simulink model "Simple_3_Model"  (R2022a)
settings: Solver=FixedStepAuto  StartTime=0.0  StopTime=10  FixedStep=.01  RelTol=1e-3
undefined symbols (not defined in the file or in its folder): importedData, robot_Volume, robotCoB, robotCoM, robotMoI, robotPitchDragCoefficients, robotRollDragCoefficients, robotXDragCoefficients, robotYawDragCoefficients, robotYDragCoefficients, robotZDragCoefficients
libraries: matrix_library x9, realtime_pacer_lib x1, ros2lib x1
settings Model: Creator=hollis  LastModifiedBy=hollis

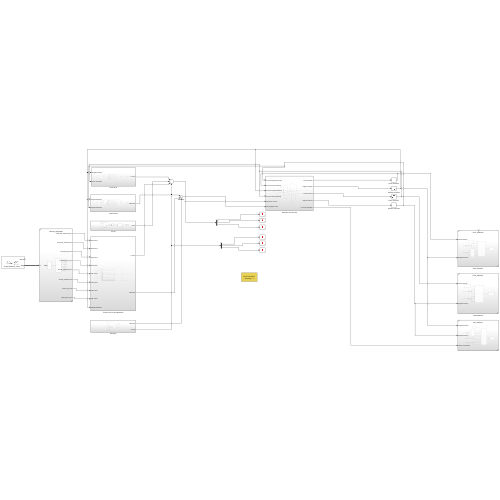
[thumbnail: Simulink's stored preview of the top-level diagram]
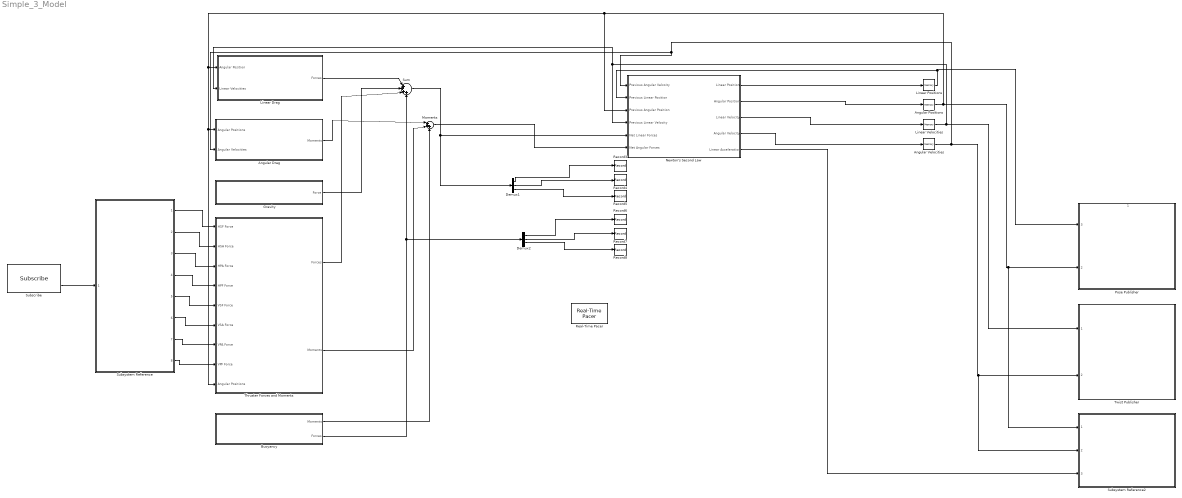
== system Simple_3_Model ==
  Angular Drag : Subsystem
  Angular Positions : Memory
  Angular Velocities : Memory
  Buoyancy : Subsystem
  Demux1 : Demux  Outputs=3
  Demux2 : Demux  Outputs=3
  Gravity : Subsystem
  Linear Drag : Subsystem
  Linear Positions : Memory
  Linear Velocities : Memory
  Moments : Sum  Inputs=|+++
  Newton's Second Law : Subsystem
  Pose Publisher : Subsystem  ReferencedSubsystem=Pose_Publisher
      settings: PortSchema="{\"entries\":[{\"content\":{\"sides\":[{\"content\":{\"connectorIds\":[\"In3\",\"In2\"]},\"type\":\"ConnectorPlacement.EquallySpacedRectSide\",\"uuid\":\"18965d15-4955-4736-88eb-98a03933ea40\"},{\"content\":{\"connectorIds\":[],\"side\":\"RIGHT\"},\"type\":\"ConnectorPlacement.EquallySpacedRectSide\",\"uuid\":\"0239975c-7916-4f79-8798-13edb7247875\"},{\"content\":{\"connectorIds\":[\"In1\"],\"side\":\"TOP\"},\"type\":\"ConnectorPlacement.EquallySpacedRectSide\",\"uuid\":\"c7399201-5872-4101-b484-2a6e35d6576e\"}]},\"type\":\"ConnectorPlacement.EquallySpacedConnector\",\"uuid\":\"5ae7f81e-60af-4dbc-8d3d-d59049f94250\"}],\"packageUris\":[\"http://schema.mathworks.com/mf0/Connector/R2020b\"],\"version\":\"1.0\"}"
  Real-Time Pacer : realtime_pacer_lib/Real-Time Pacer  simTimePerRealTime=1
      settings: SourceProductName=Real-Time Pacer
  Record3 : Record  FileSettingsInternal="{\"entries\":[{\"content\":{\"excelSettings\":{\"content\":{},\"type\":\"Streamout.ExcelSettings\"}},\"type\":\"Streamout.FileSettingStorage\",\"uuid\":\"7fd3eebb-0f88-428b-bc5a-be43bf9f2e21\"}],\"packageUris\":[\"http://schema.mathworks.com/mf0/streamout_blocks/R2020a\"],\"version\":\"1.0\"}"  SignalsInternal="{\"entries\":[{\"content\":{\"signals\":[{\"content\":{\"blockPath\":[\"Simple_3_Model/Record3\"],\"channel\":[],\"dimensions\":[1,1],\"domain\":\"Simple_3_Model/Record3\",\"lineColor\":\"#4dbeee\",\"plots\":[1],\"port\":1,\"sid\":[\"\"],\"signalID\":351,\"signalName\":\"Demux1:1\"},\"type\":\"RecordBlkView.Signal\",\"uuid\":\"b88f4a68-92d4-4a9b-a347-9b0300d270aa\"}]},\"type\":\"RecordBlkView.InputSignals\",\"uuid\":\"525ea289-2c7b-4200-a763-2aaae37b50f9\"}],\"packageUris\":[\"http://schema.mathworks.com/mf0/streamout_blocks/R2020a\"],\"version\":\"1.0\"}"  VisualizationBindings="{\"sparklinesplugin\":{\"info\":[{\"bindingParametersList\":[],\"subplotID\":1}]}}"
  Record4 : Record  FileSettingsInternal="{\"entries\":[{\"content\":{\"excelSettings\":{\"content\":{},\"type\":\"Streamout.ExcelSettings\"}},\"type\":\"Streamout.FileSettingStorage\",\"uuid\":\"25a64ef7-4cd6-46f5-99bd-b94f42d1ee70\"}],\"packageUris\":[\"http://schema.mathworks.com/mf0/streamout_blocks/R2020a\"],\"version\":\"1.0\"}"  SignalsInternal="{\"entries\":[{\"content\":{\"signals\":[{\"content\":{\"blockPath\":[\"Simple_3_Model/Record4\"],\"channel\":[],\"dimensions\":[1,1],\"domain\":\"Simple_3_Model/Record4\",\"lineColor\":\"#a2142f\",\"plots\":[1],\"port\":1,\"sid\":[\"\"],\"signalID\":355,\"signalName\":\"Demux1:2\"},\"type\":\"RecordBlkView.Signal\",\"uuid\":\"ab564040-d490-4015-8163-6bd6843044f3\"}]},\"type\":\"RecordBlkView.InputSignals\",\"uuid\":\"276f9bd8-9c59-4519-84f4-c5845e1178bb\"}],\"packageUris\":[\"http://schema.mathworks.com/mf0/streamout_blocks/R2020a\"],\"version\":\"1.0\"}"  VisualizationBindings="{\"sparklinesplugin\":{\"info\":[{\"bindingParametersList\":[],\"subplotID\":1}]}}"
  Record5 : Record  FileSettingsInternal="{\"entries\":[{\"content\":{\"excelSettings\":{\"content\":{},\"type\":\"Streamout.ExcelSettings\"}},\"type\":\"Streamout.FileSettingStorage\",\"uuid\":\"6c523934-be1b-4723-a5da-1a53bd07d317\"}],\"packageUris\":[\"http://schema.mathworks.com/mf0/streamout_blocks/R2020a\"],\"version\":\"1.0\"}"  SignalsInternal="{\"entries\":[{\"content\":{\"signals\":[{\"content\":{\"blockPath\":[\"Simple_3_Model/Record5\"],\"channel\":[],\"dimensions\":[1,1],\"domain\":\"Simple_3_Model/Record5\",\"lineColor\":\"#139fff\",\"plots\":[1],\"port\":1,\"sid\":[\"\"],\"signalID\":359,\"signalName\":\"Demux1:3\"},\"type\":\"RecordBlkView.Signal\",\"uuid\":\"c0e7c173-a5c9-49b7-9f71-2d8dfa5ec17e\"}]},\"type\":\"RecordBlkView.InputSignals\",\"uuid\":\"c924540a-dae3-4e11-a7aa-2d2acfbdbe16\"}],\"packageUris\":[\"http://schema.mathworks.com/mf0/streamout_blocks/R2020a\"],\"version\":\"1.0\"}"  VisualizationBindings="{\"sparklinesplugin\":{\"info\":[{\"bindingParametersList\":[],\"subplotID\":1}]}}"
  Record6 : Record  FileSettingsInternal="{\"entries\":[{\"content\":{\"excelSettings\":{\"content\":{},\"type\":\"Streamout.ExcelSettings\"}},\"type\":\"Streamout.FileSettingStorage\",\"uuid\":\"7e9df886-1170-419d-9cbc-cbe48d003bf2\"}],\"packageUris\":[\"http://schema.mathworks.com/mf0/streamout_blocks/R2020a\"],\"version\":\"1.0\"}"  SignalsInternal="{\"entries\":[{\"content\":{\"signals\":[{\"content\":{\"blockPath\":[\"Simple_3_Model/Record6\"],\"channel\":[],\"dimensions\":[1,1],\"domain\":\"Simple_3_Model/Record6\",\"lineColor\":\"#edb120\",\"plots\":[1],\"port\":1,\"sid\":[\"\"],\"signalID\":363,\"signalName\":\"Demux2:1\"},\"type\":\"RecordBlkView.Signal\",\"uuid\":\"9d71cc72-7893-4320-bde5-368aaa6a6399\"}]},\"type\":\"RecordBlkView.InputSignals\",\"uuid\":\"6ba886b7-fc5d-4a52-a6dc-8621a5dc22ea\"}],\"packageUris\":[\"http://schema.mathworks.com/mf0/streamout_blocks/R2020a\"],\"version\":\"1.0\"}"  VisualizationBindings="{\"sparklinesplugin\":{\"info\":[{\"bindingParametersList\":[],\"subplotID\":1}]}}"
  Record7 : Record  FileSettingsInternal="{\"entries\":[{\"content\":{\"excelSettings\":{\"content\":{},\"type\":\"Streamout.ExcelSettings\"}},\"type\":\"Streamout.FileSettingStorage\",\"uuid\":\"db813548-beb3-4592-95ed-07357187fff0\"}],\"packageUris\":[\"http://schema.mathworks.com/mf0/streamout_blocks/R2020a\"],\"version\":\"1.0\"}"  SignalsInternal="{\"entries\":[{\"content\":{\"signals\":[{\"content\":{\"blockPath\":[\"Simple_3_Model/Record7\"],\"channel\":[],\"dimensions\":[1,1],\"domain\":\"Simple_3_Model/Record7\",\"lineColor\":\"#7e2f8e\",\"plots\":[1],\"port\":1,\"sid\":[\"\"],\"signalID\":367,\"signalName\":\"Demux2:2\"},\"type\":\"RecordBlkView.Signal\",\"uuid\":\"a9a06697-73f9-436b-bc11-ccf928b186fe\"}]},\"type\":\"RecordBlkView.InputSignals\",\"uuid\":\"18b6c55c-c8ab-460b-beea-45484844a1c5\"}],\"packageUris\":[\"http://schema.mathworks.com/mf0/streamout_blocks/R2020a\"],\"version\":\"1.0\"}"  VisualizationBindings="{\"sparklinesplugin\":{\"info\":[{\"bindingParametersList\":[],\"subplotID\":1}]}}"
  Record8 : Record  FileSettingsInternal="{\"entries\":[{\"content\":{\"excelSettings\":{\"content\":{},\"type\":\"Streamout.ExcelSettings\"}},\"type\":\"Streamout.FileSettingStorage\",\"uuid\":\"193b8698-55d3-4337-bca1-470059843305\"}],\"packageUris\":[\"http://schema.mathworks.com/mf0/streamout_blocks/R2020a\"],\"version\":\"1.0\"}"  SignalsInternal="{\"entries\":[{\"content\":{\"signals\":[{\"content\":{\"blockPath\":[\"Simple_3_Model/Record8\"],\"channel\":[],\"dimensions\":[1,1],\"domain\":\"Simple_3_Model/Record8\",\"lineColor\":\"#77ac30\",\"plots\":[1],\"port\":1,\"sid\":[\"\"],\"signalID\":371,\"signalName\":\"Demux2:3\"},\"type\":\"RecordBlkView.Signal\",\"uuid\":\"1c0420e5-8b4b-4d3a-992d-29d5925925d9\"}]},\"type\":\"RecordBlkView.InputSignals\",\"uuid\":\"2ac1f8f1-2e48-4e86-bbdb-ec48a12e78c2\"}],\"packageUris\":[\"http://schema.mathworks.com/mf0/streamout_blocks/R2020a\"],\"version\":\"1.0\"}"  VisualizationBindings="{\"sparklinesplugin\":{\"info\":[{\"bindingParametersList\":[],\"subplotID\":1}]}}"
  Subscribe : ros2lib/Subscribe  topicSource=Select from ROS network  topic=/tempest/thruster_forces  messageType=std_msgs/Float32MultiArray  sampleTime=-1  QOSHistory=Keep last  QOSDepth=1  QOSReliability=Reliable  QOSDurability=Volatile
      settings: SourceProductBaseCode=RR
  Subsystem Reference : Subsystem  ReferencedSubsystem=Thruster_Magnitude
  Subsystem Reference2 : Subsystem  ReferencedSubsystem=Imu_Publisher
  Sum : Sum  Inputs=|++++
  Thruster Forces and Moments : Subsystem
  Twist Publisher : Subsystem  ReferencedSubsystem=Twist_Publisher
  wires:
  Linear Drag/1(Forces) -> Sum/1
  Gravity/1(Force) -> Sum/2
  Angular Drag/1(Moments) -> Moments/1
  Thruster Forces and Moments/2(Moments) -> Moments/2
  Buoyancy/1(Moments) -> Moments/3
  Angular Velocities/1 -> Subsystem Reference2/2, Twist Publisher/2, Angular Drag/2(Angular Velocities), Newton's Second Law/1(Previous Angular Velcoity)
  Linear Positions/1 -> Pose Publisher/3, Newton's Second Law/2(Previous Linear Position)
  Linear Velocities/1 -> Linear Drag/2(Linear Velocities), Newton's Second Law/4(Previous Linear Velocity), Twist Publisher/1
  Sum/1 -> Demux1/1, Newton's Second Law/5(Net Linear Forces)
  Moments/1 -> Newton's Second Law/6(Net Angular Forces)
  Newton's Second Law/1(Linear Position) -> Linear Positions/1
  Newton's Second Law/2(Angular Position) -> Angular Positions/1
  Newton's Second Law/4(Angular Velocity) -> Angular Velocities/1
  Newton's Second Law/3(Linear Velocity) -> Linear Velocities/1
  Angular Positions/1 -> Linear Drag/1(Angular Position), Thruster Forces and Moments/9(Angular Positions), Angular Drag/1(Angular Positions), Newton's Second Law/3(Previous Angular Position), Subsystem Reference2/1, Pose Publisher/2
  Demux1/2 -> Record4/1
  Demux1/1 -> Record3/1
  Demux1/3 -> Record5/1
  Thruster Forces and Moments/1(Forces) -> Sum/3
  Demux2/2 -> Record7/1
  Demux2/1 -> Record6/1
  Demux2/3 -> Record8/1
  Buoyancy/2(Forces) -> Sum/4, Demux2/1
  Subsystem Reference/1 -> Thruster Forces and Moments/1(HSF Force)
  Subsystem Reference/2 -> Thruster Forces and Moments/2(HSA Force)
  Subsystem Reference/3 -> Thruster Forces and Moments/3(HPA Force)
  Subsystem Reference/4 -> Thruster Forces and Moments/4(HPF Force)
  Subsystem Reference/5 -> Thruster Forces and Moments/5(VSF Force)
  Subsystem Reference/6 -> Thruster Forces and Moments/6(VSA Force)
  Subsystem Reference/7 -> Thruster Forces and Moments/7(VPA Force)
  Subsystem Reference/8 -> Thruster Forces and Moments/8(VPF Force)
  Subscribe/2 -> Subsystem Reference/1
  Newton's Second Law/5(Linear Acceleration) -> Subsystem Reference2/3

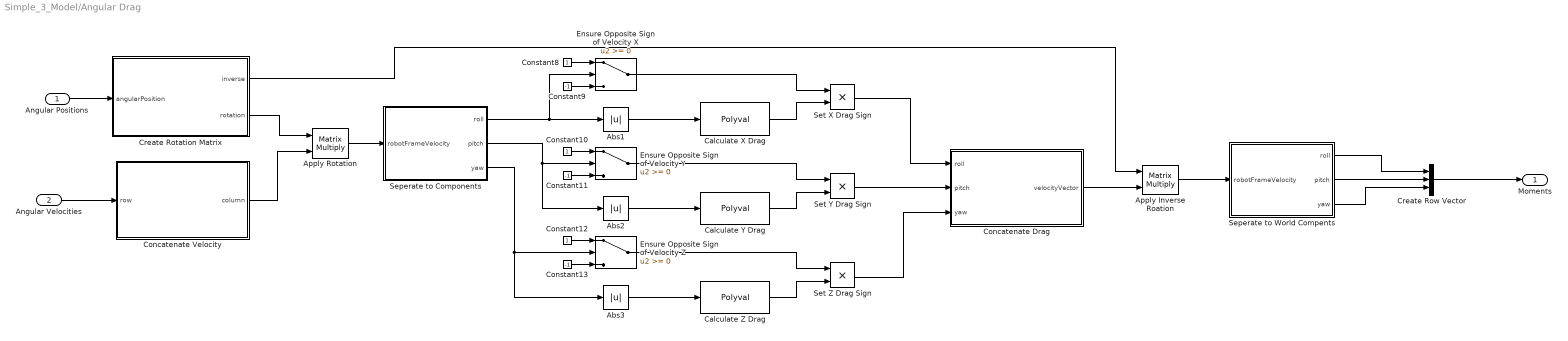
== system Simple_3_Model/Angular Drag ==
  Angular Positions : Inport
  Angular Velocities : Inport  Port=2
  Abs1 : Abs  SaturateOnIntegerOverflow=off
  Abs2 : Abs  SaturateOnIntegerOverflow=off
  Abs3 : Abs  SaturateOnIntegerOverflow=off
  Apply Inverse Roation : Product  Multiplication=Matrix(*)
  Apply Rotation : Product  Multiplication=Matrix(*)
  Calculate X Drag : Polyval  Coefs=robotRollDragCoefficients
  Calculate Y Drag : Polyval  Coefs=robotPitchDragCoefficients
  Calculate Z Drag : Polyval  Coefs=robotYawDragCoefficients
  Concatenate Drag : MATLAB Function  TreatAsAtomicUnit=on
  Concatenate Velocity : MATLAB Function  TreatAsAtomicUnit=on
  Constant10 : Constant
  Constant11 : Constant  Value=-1
  Constant12 : Constant
  Constant13 : Constant  Value=-1
  Constant8 : Constant
  Constant9 : Constant  Value=-1
  Create Rotation Matrix : MATLAB Function  TreatAsAtomicUnit=on
  Create Row Vector : Mux  Inputs=3
  Ensure Opposite Sign of Velocity X : Switch  SaturateOnIntegerOverflow=off  InputSameDT=off
  Ensure Opposite Sign of Velocity Y : Switch  SaturateOnIntegerOverflow=off  InputSameDT=off
  Ensure Opposite Sign of Velocity Z : Switch  SaturateOnIntegerOverflow=off  InputSameDT=off
  Seperate to Components : MATLAB Function  TreatAsAtomicUnit=on
  Seperate to World Compents : MATLAB Function  TreatAsAtomicUnit=on
  Set X Drag Sign : Product
  Set Y Drag Sign : Product
  Set Z Drag Sign : Product
  Moments : Outport
  wires:
  Concatenate Drag/1(velocityVector) -> Apply Inverse Roation/2
  Calculate Y Drag/1 -> Set Y Drag Sign/2
  Constant11/1 -> Ensure Opposite Sign of Velocity Y/3
  Calculate Z Drag/1 -> Set Z Drag Sign/2
  Abs1/1 -> Calculate X Drag/1
  Apply Rotation/1 -> Seperate to Components/1(robotFrameVelocity)
  Apply Inverse Roation/1 -> Seperate to World Compents/1(robotFrameVelocity)
  Angular Velocities/1 -> Concatenate Velocity/1(row)
  Constant8/1 -> Ensure Opposite Sign of Velocity X/1
  Set Z Drag Sign/1 -> Concatenate Drag/3(yaw)
  Constant13/1 -> Ensure Opposite Sign of Velocity Z/3
  Constant9/1 -> Ensure Opposite Sign of Velocity X/3
  Set Y Drag Sign/1 -> Concatenate Drag/2(pitch)
  Ensure Opposite Sign of Velocity Y/1 -> Set Y Drag Sign/1
  Seperate to Components/2(pitch) -> Abs2/1, Ensure Opposite Sign of Velocity Y/2
  Set X Drag Sign/1 -> Concatenate Drag/1(roll)
  Seperate to World Compents/3(yaw) -> Create Row Vector/3
  Constant12/1 -> Ensure Opposite Sign of Velocity Z/1
  Create Rotation Matrix/2(rotation) -> Apply Rotation/1
  Concatenate Velocity/1(column) -> Apply Rotation/2
  Seperate to World Compents/1(roll) -> Create Row Vector/1
  Ensure Opposite Sign of Velocity X/1 -> Set X Drag Sign/1
  Seperate to Components/1(roll) -> Ensure Opposite Sign of Velocity X/2, Abs1/1
  Seperate to World Compents/2(pitch) -> Create Row Vector/2
  Create Rotation Matrix/1(inverse) -> Apply Inverse Roation/1
  Constant10/1 -> Ensure Opposite Sign of Velocity Y/1
  Calculate X Drag/1 -> Set X Drag Sign/2
  Abs2/1 -> Calculate Y Drag/1
  Abs3/1 -> Calculate Z Drag/1
  Seperate to Components/3(yaw) -> Ensure Opposite Sign of Velocity Z/2, Abs3/1
  Ensure Opposite Sign of Velocity Z/1 -> Set Z Drag Sign/1
  Create Row Vector/1 -> Moments/1
  Angular Positions/1 -> Create Rotation Matrix/1(angularPosition)

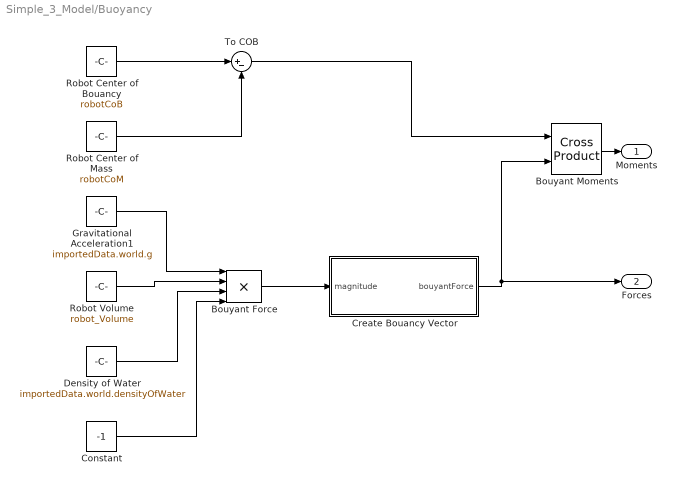
== system Simple_3_Model/Buoyancy ==
  Bouyant Force : Product  Inputs=4
  Bouyant Moments : matrix_library/Cross Product
      settings: SourceProductBaseCode=SL
  Constant : Constant  Value=-1
  Create Bouancy Vector : MATLAB Function  TreatAsAtomicUnit=on
  Density of Water : Constant  Value=importedData.world.densityOfWater
  Gravitational Acceleration1 : Constant  Value=importedData.world.g
  Robot Center of Bouancy : Constant  Value=robotCoB
  Robot Center of Mass : Constant  Value=robotCoM
  Robot Volume : Constant  Value=robot_Volume
  To COB : Sum  Inputs=|+-
  Moments : Outport
  Forces : Outport  Port=2
  wires:
  Density of Water/1 -> Bouyant Force/3
  Gravitational Acceleration1/1 -> Bouyant Force/1
  Robot Center of Bouancy/1 -> To COB/1
  To COB/1 -> Bouyant Moments/1
  Bouyant Force/1 -> Create Bouancy Vector/1(magnitude)
  Create Bouancy Vector/1(bouyantForce) -> Bouyant Moments/2, Forces/1
  Robot Volume/1 -> Bouyant Force/2
  Robot Center of Mass/1 -> To COB/2
  Bouyant Moments/1 -> Moments/1
  Constant/1 -> Bouyant Force/4

== system Simple_3_Model/Gravity ==
  Create Vector : MATLAB Function  TreatAsAtomicUnit=on
  Gravitational Acceleration1 : Constant  Value=importedData.world.g
  Gravitational Force1 : Product
  Robot Mass : Constant  Value=33.5
  Force : Outport
  wires:
  Gravitational Acceleration1/1 -> Gravitational Force1/1
  Robot Mass/1 -> Gravitational Force1/2
  Create Vector/1(vector) -> Force/1
  Gravitational Force1/1 -> Create Vector/1(magnitude)

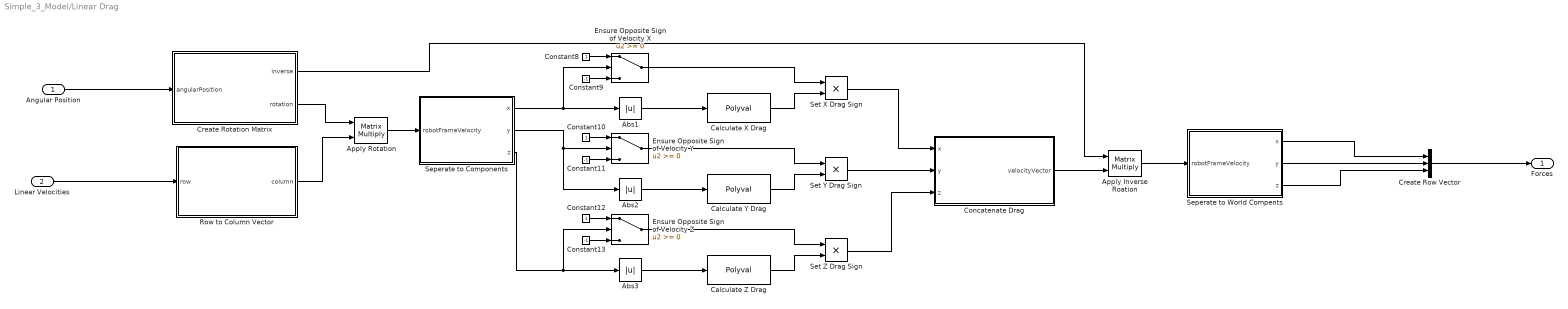
== system Simple_3_Model/Linear Drag ==
  Angular Position : Inport
  Linear Velocities : Inport  Port=2
  Abs1 : Abs  SaturateOnIntegerOverflow=off
  Abs2 : Abs  SaturateOnIntegerOverflow=off
  Abs3 : Abs  SaturateOnIntegerOverflow=off
  Apply Inverse Roation : Product  Multiplication=Matrix(*)
  Apply Rotation : Product  Multiplication=Matrix(*)
  Calculate X Drag : Polyval  Coefs=robotXDragCoefficients
  Calculate Y Drag : Polyval  Coefs=robotYDragCoefficients
  Calculate Z Drag : Polyval  Coefs=robotZDragCoefficients
  Concatenate Drag : MATLAB Function  TreatAsAtomicUnit=on
  Constant10 : Constant
  Constant11 : Constant  Value=-1
  Constant12 : Constant
  Constant13 : Constant  Value=-1
  Constant8 : Constant
  Constant9 : Constant  Value=-1
  Create Rotation Matrix : MATLAB Function  TreatAsAtomicUnit=on
  Create Row Vector : Mux  Inputs=3
  Ensure Opposite Sign of Velocity X : Switch  SaturateOnIntegerOverflow=off  InputSameDT=off
  Ensure Opposite Sign of Velocity Y : Switch  SaturateOnIntegerOverflow=off  InputSameDT=off
  Ensure Opposite Sign of Velocity Z : Switch  SaturateOnIntegerOverflow=off  InputSameDT=off
  Row to Column Vector : MATLAB Function  TreatAsAtomicUnit=on
  Seperate to Components : MATLAB Function  TreatAsAtomicUnit=on
  Seperate to World Compents : MATLAB Function  TreatAsAtomicUnit=on
  Set X Drag Sign : Product
  Set Y Drag Sign : Product
  Set Z Drag Sign : Product
  Forces : Outport
  wires:
  Calculate X Drag/1 -> Set X Drag Sign/2
  Ensure Opposite Sign of Velocity X/1 -> Set X Drag Sign/1
  Constant12/1 -> Ensure Opposite Sign of Velocity Z/1
  Abs2/1 -> Calculate Y Drag/1
  Constant8/1 -> Ensure Opposite Sign of Velocity X/1
  Seperate to Components/3(z) -> Abs3/1, Ensure Opposite Sign of Velocity Z/2
  Set Z Drag Sign/1 -> Concatenate Drag/3(z)
  Abs3/1 -> Calculate Z Drag/1
  Abs1/1 -> Calculate X Drag/1
  Concatenate Drag/1(velocityVector) -> Apply Inverse Roation/2
  Calculate Y Drag/1 -> Set Y Drag Sign/2
  Apply Inverse Roation/1 -> Seperate to World Compents/1(robotFrameVelocity)
  Constant9/1 -> Ensure Opposite Sign of Velocity X/3
  Constant13/1 -> Ensure Opposite Sign of Velocity Z/3
  Create Rotation Matrix/1(inverse) -> Apply Inverse Roation/1
  Create Rotation Matrix/2(rotation) -> Apply Rotation/1
  Row to Column Vector/1(column) -> Apply Rotation/2
  Constant10/1 -> Ensure Opposite Sign of Velocity Y/1
  Seperate to Components/2(y) -> Abs2/1, Ensure Opposite Sign of Velocity Y/2
  Seperate to Components/1(x) -> Abs1/1, Ensure Opposite Sign of Velocity X/2
  Constant11/1 -> Ensure Opposite Sign of Velocity Y/3
  Apply Rotation/1 -> Seperate to Components/1(robotFrameVelocity)
  Calculate Z Drag/1 -> Set Z Drag Sign/2
  Angular Position/1 -> Create Rotation Matrix/1(angularPosition)
  Ensure Opposite Sign of Velocity Y/1 -> Set Y Drag Sign/1
  Set Y Drag Sign/1 -> Concatenate Drag/2(y)
  Set X Drag Sign/1 -> Concatenate Drag/1(x)
  Ensure Opposite Sign of Velocity Z/1 -> Set Z Drag Sign/1
  Seperate to World Compents/2(y) -> Create Row Vector/2
  Seperate to World Compents/1(x) -> Create Row Vector/1
  Seperate to World Compents/3(z) -> Create Row Vector/3
  Create Row Vector/1 -> Forces/1
  Linear Velocities/1 -> Row to Column Vector/1(row)

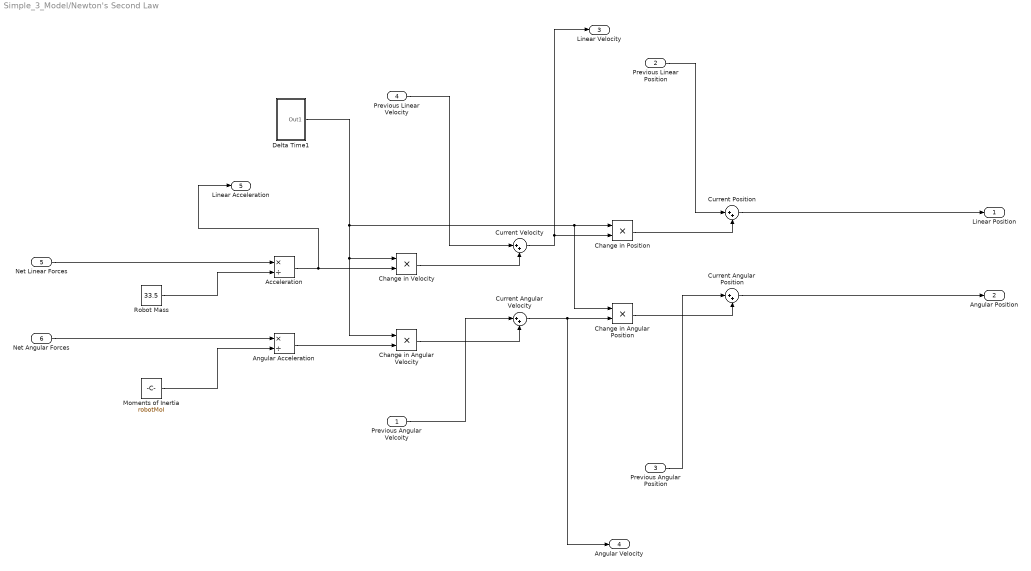
== system Simple_3_Model/Newton's Second Law ==
  Previous Angular Velcoity : Inport
  Previous Linear Position : Inport  Port=2
  Previous Angular Position : Inport  Port=3
  Previous Linear Velocity : Inport  Port=4
  Net Linear Forces : Inport  Port=5
  Net Angular Forces : Inport  Port=6
  Acceleration : Product  Inputs=*/
  Angular Acceleration : Product  Inputs=*/
  Change in Angular Position : Product
  Change in Angular Velocity : Product
  Change in Position : Product
  Change in Velocity : Product
  Current Angular Position : Sum  Inputs=|++
  Current Angular Velocity : Sum  Inputs=|++
  Current Position : Sum  Inputs=|++
  Current Velocity : Sum  Inputs=|++
  Delta Time1 : Subsystem
  Moments of Inertia : Constant  Value=robotMoI
  Robot Mass : Constant  Value=33.5
  Linear Position : Outport
  Angular Position : Outport  Port=2
  Linear Velocity : Outport  Port=3
  Angular Velocity : Outport  Port=4
  Linear Acceleration : Outport  Port=5
  wires:
  Current Angular Position/1 -> Angular Position/1
  Acceleration/1 -> Linear Acceleration/1, Change in Velocity/2
  Angular Acceleration/1 -> Change in Angular Velocity/2
  Change in Position/1 -> Current Position/2
  Moments of Inertia/1 -> Angular Acceleration/2
  Current Velocity/1 -> Linear Velocity/1, Change in Position/2
  Current Position/1 -> Linear Position/1
  Previous Linear Velocity/1 -> Current Velocity/1
  Change in Angular Velocity/1 -> Current Angular Velocity/2
  Net Linear Forces/1 -> Acceleration/1
  Net Angular Forces/1 -> Angular Acceleration/1
  Current Angular Velocity/1 -> Angular Velocity/1, Change in Angular Position/2
  Change in Angular Position/1 -> Current Angular Position/2
  Previous Angular Velcoity/1 -> Current Angular Velocity/1
  Delta Time1/1(Out1) -> Change in Angular Velocity/1, Change in Velocity/1, Change in Angular Position/1, Change in Position/1
  Previous Linear Position/1 -> Current Position/1
  Robot Mass/1 -> Acceleration/2
  Previous Angular Position/1 -> Current Angular Position/1
  Change in Velocity/1 -> Current Velocity/2

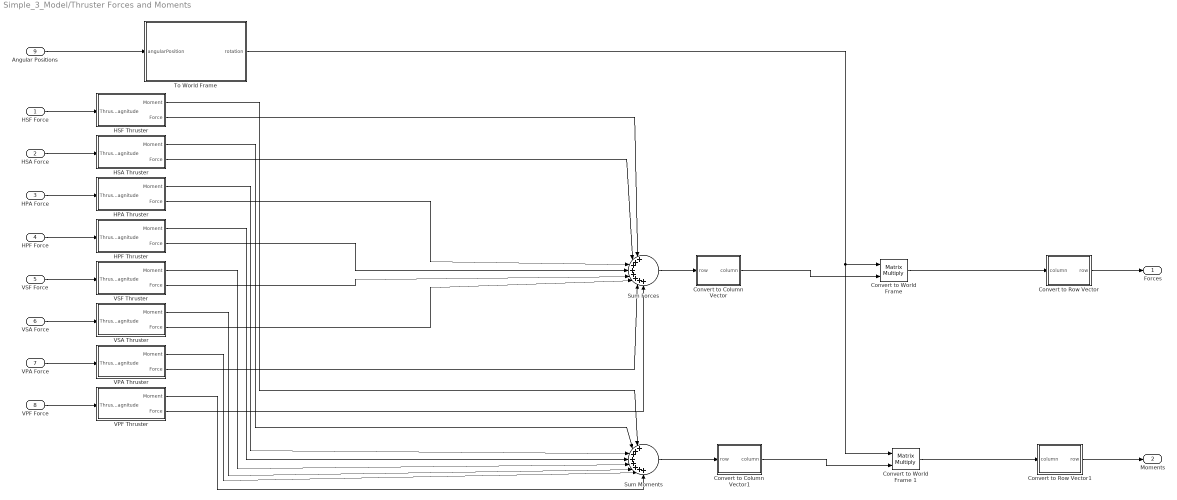
== system Simple_3_Model/Thruster Forces and Moments ==
  HSF Force : Inport
  HSA Force : Inport  Port=2
  HPA Force : Inport  Port=3
  HPF Force : Inport  Port=4
  VSF Force : Inport  Port=5
  VSA Force : Inport  Port=6
  VPA Force : Inport  Port=7
  VPF Force : Inport  Port=8
  Angular Positions : Inport  Port=9
  Convert to Column Vector : MATLAB Function  TreatAsAtomicUnit=on
  Convert to Column Vector1 : MATLAB Function  TreatAsAtomicUnit=on
  Convert to Row Vector : MATLAB Function  TreatAsAtomicUnit=on
  Convert to Row Vector1 : MATLAB Function  TreatAsAtomicUnit=on
  Convert to World Frame : Product  Multiplication=Matrix(*)
  Convert to World Frame 1 : Product  Multiplication=Matrix(*)
  HPA Thruster : Subsystem
  HPF Thruster : Subsystem
  HSA Thruster : Subsystem
  HSF Thruster : Subsystem
  Sum Forces : Sum  Inputs=|++++++++  InputSameDT=on
  Sum Moments : Sum  Inputs=|++++++++
  To World Frame : MATLAB Function  TreatAsAtomicUnit=on
  VPA Thruster : Subsystem
  VPF Thruster : Subsystem
  VSA Thruster : Subsystem
  VSF Thruster : Subsystem
  Forces : Outport
  Moments : Outport  Port=2
  wires:
  VSF Thruster/2(Force) -> Sum Forces/5
  HSF Thruster/1(Moment) -> Sum Moments/1
  HSF Force/1 -> HSF Thruster/1(Thrust Magnitude)
  VSF Thruster/1(Moment) -> Sum Moments/5
  HPA Thruster/1(Moment) -> Sum Moments/3
  VSF Force/1 -> VSF Thruster/1(Thrust Magnitude)
  HPF Thruster/2(Force) -> Sum Forces/4
  HSA Thruster/1(Moment) -> Sum Moments/2
  VSA Thruster/2(Force) -> Sum Forces/6
  HPF Thruster/1(Moment) -> Sum Moments/4
  VPA Force/1 -> VPA Thruster/1(Thrust Magnitude)
  VPF Force/1 -> VPF Thruster/1(Thrust Magnitude)
  VPF Thruster/1(Moment) -> Sum Moments/8
  HSA Thruster/2(Force) -> Sum Forces/2
  VSA Force/1 -> VSA Thruster/1(Thrust Magnitude)
  HPF Force/1 -> HPF Thruster/1(Thrust Magnitude)
  VPA Thruster/2(Force) -> Sum Forces/7
  HPA Thruster/2(Force) -> Sum Forces/3
  Sum Forces/1 -> Convert to Column Vector/1(row)
  HSF Thruster/2(Force) -> Sum Forces/1
  HPA Force/1 -> HPA Thruster/1(Thrust Magnitude)
  VPA Thruster/1(Moment) -> Sum Moments/7
  HSA Force/1 -> HSA Thruster/1(Thrust Magnitude)
  VPF Thruster/2(Force) -> Sum Forces/8
  VSA Thruster/1(Moment) -> Sum Moments/6
  Angular Positions/1 -> To World Frame/1(angularPosition)
  Convert to Row Vector/1(row) -> Forces/1
  Convert to Column Vector/1(column) -> Convert to World Frame/2
  Convert to World Frame/1 -> Convert to Row Vector/1(column)
  To World Frame/1(rotation) -> Convert to World Frame 1/1, Convert to World Frame/1
  Convert to World Frame 1/1 -> Convert to Row Vector1/1(column)
  Convert to Row Vector1/1(row) -> Moments/1
  Convert to Column Vector1/1(column) -> Convert to World Frame 1/2
  Sum Moments/1 -> Convert to Column Vector1/1(row)

== system Simple_3_Model/Newton's Second Law/Delta Time1 ==
  Clock : Clock
  Delta Time : Sum  Inputs=|+-
  Memory1 : Memory
  Out1 : Outport
  wires:
  Memory1/1 -> Delta Time/2
  Clock/1 -> Memory1/1, Delta Time/1
  Delta Time/1 -> Out1/1

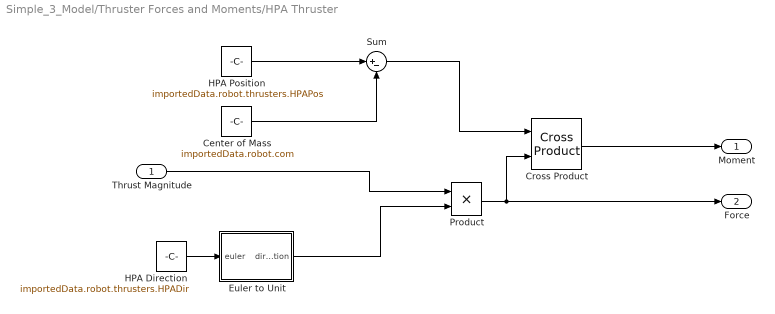
== system Simple_3_Model/Thruster Forces and Moments/HPA Thruster ==
  Thrust Magnitude : Inport
  Center of Mass : Constant  Value=importedData.robot.com
  Cross Product : matrix_library/Cross Product
      settings: SourceProductBaseCode=SL
  Euler to Unit : MATLAB Function  TreatAsAtomicUnit=on
  HPA Direction : Constant  Value=importedData.robot.thrusters.HPADir  VectorParams1D=off
  HPA Position : Constant  Value=importedData.robot.thrusters.HPAPos  VectorParams1D=off
  Product : Product
  Sum : Sum  Inputs=|+-
  Moment : Outport
  Force : Outport  Port=2
  wires:
  Product/1 -> Force/1, Cross Product/2
  Cross Product/1 -> Moment/1
  Thrust Magnitude/1 -> Product/1
  HPA Direction/1 -> Euler to Unit/1(euler)
  Euler to Unit/1(direction) -> Product/2
  HPA Position/1 -> Sum/1
  Center of Mass/1 -> Sum/2
  Sum/1 -> Cross Product/1

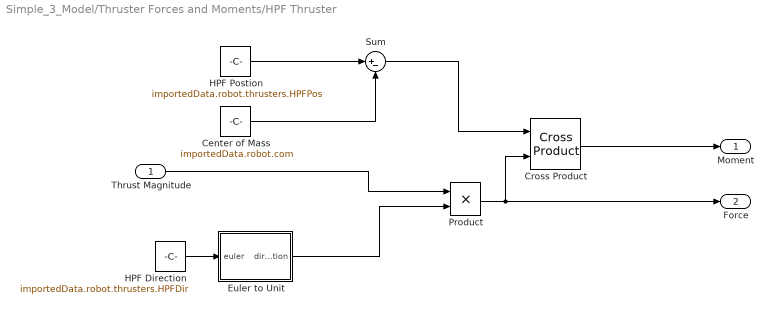
== system Simple_3_Model/Thruster Forces and Moments/HPF Thruster ==
  Thrust Magnitude : Inport
  Center of Mass : Constant  Value=importedData.robot.com
  Cross Product : matrix_library/Cross Product
      settings: SourceProductBaseCode=SL
  Euler to Unit : MATLAB Function  TreatAsAtomicUnit=on
  HPF Direction : Constant  Value=importedData.robot.thrusters.HPFDir  VectorParams1D=off
  HPF Postion : Constant  Value=importedData.robot.thrusters.HPFPos  VectorParams1D=off
  Product : Product
  Sum : Sum  Inputs=|+-
  Moment : Outport
  Force : Outport  Port=2
  wires:
  Product/1 -> Force/1, Cross Product/2
  Cross Product/1 -> Moment/1
  Thrust Magnitude/1 -> Product/1
  HPF Direction/1 -> Euler to Unit/1(euler)
  Euler to Unit/1(direction) -> Product/2
  HPF Postion/1 -> Sum/1
  Center of Mass/1 -> Sum/2
  Sum/1 -> Cross Product/1

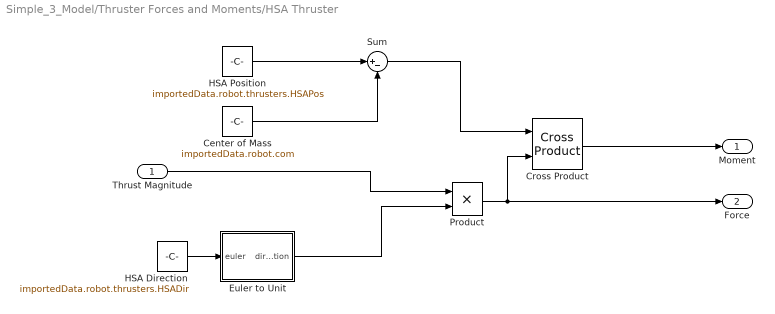
== system Simple_3_Model/Thruster Forces and Moments/HSA Thruster ==
  Thrust Magnitude : Inport
  Center of Mass : Constant  Value=importedData.robot.com
  Cross Product : matrix_library/Cross Product
      settings: SourceProductBaseCode=SL
  Euler to Unit : MATLAB Function  TreatAsAtomicUnit=on
  HSA Direction : Constant  Value=importedData.robot.thrusters.HSADir  VectorParams1D=off
  HSA Position : Constant  Value=importedData.robot.thrusters.HSAPos  VectorParams1D=off
  Product : Product
  Sum : Sum  Inputs=|+-
  Moment : Outport
  Force : Outport  Port=2
  wires:
  Product/1 -> Force/1, Cross Product/2
  Cross Product/1 -> Moment/1
  Thrust Magnitude/1 -> Product/1
  HSA Direction/1 -> Euler to Unit/1(euler)
  Euler to Unit/1(direction) -> Product/2
  HSA Position/1 -> Sum/1
  Center of Mass/1 -> Sum/2
  Sum/1 -> Cross Product/1

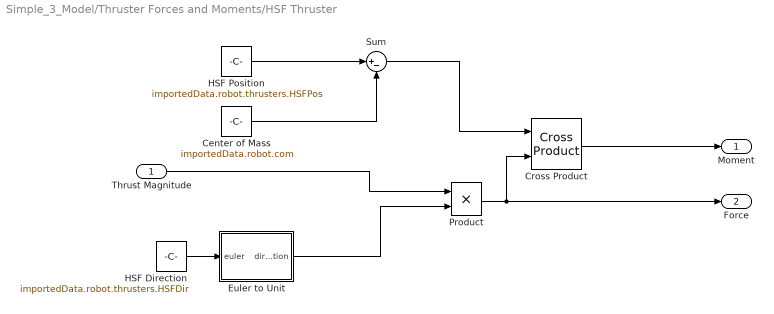
== system Simple_3_Model/Thruster Forces and Moments/HSF Thruster ==
  Thrust Magnitude : Inport
  Center of Mass : Constant  Value=importedData.robot.com
  Cross Product : matrix_library/Cross Product
      settings: SourceProductBaseCode=SL
  Euler to Unit : MATLAB Function  TreatAsAtomicUnit=on
  HSF Direction : Constant  Value=importedData.robot.thrusters.HSFDir  VectorParams1D=off
  HSF Position : Constant  Value=importedData.robot.thrusters.HSFPos  VectorParams1D=off
  Product : Product
  Sum : Sum  Inputs=|+-
  Moment : Outport
  Force : Outport  Port=2
  wires:
  Product/1 -> Force/1, Cross Product/2
  Cross Product/1 -> Moment/1
  Thrust Magnitude/1 -> Product/1
  HSF Direction/1 -> Euler to Unit/1(euler)
  Euler to Unit/1(direction) -> Product/2
  HSF Position/1 -> Sum/1
  Center of Mass/1 -> Sum/2
  Sum/1 -> Cross Product/1

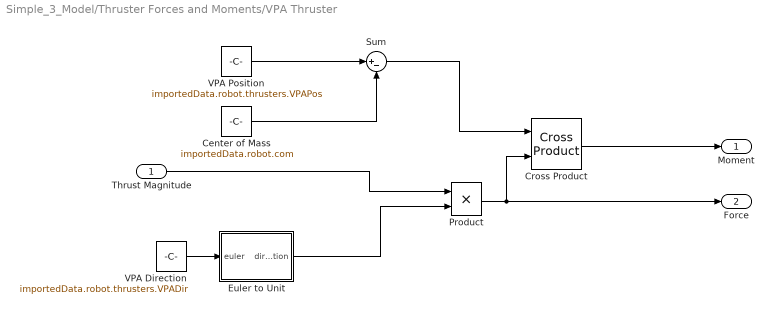
== system Simple_3_Model/Thruster Forces and Moments/VPA Thruster ==
  Thrust Magnitude : Inport
  Center of Mass : Constant  Value=importedData.robot.com
  Cross Product : matrix_library/Cross Product
      settings: SourceProductBaseCode=SL
  Euler to Unit : MATLAB Function  TreatAsAtomicUnit=on
  Product : Product
  Sum : Sum  Inputs=|+-
  VPA Direction : Constant  Value=importedData.robot.thrusters.VPADir  VectorParams1D=off
  VPA Position : Constant  Value=importedData.robot.thrusters.VPAPos  VectorParams1D=off
  Moment : Outport
  Force : Outport  Port=2
  wires:
  Product/1 -> Force/1, Cross Product/2
  Cross Product/1 -> Moment/1
  Thrust Magnitude/1 -> Product/1
  VPA Direction/1 -> Euler to Unit/1(euler)
  Euler to Unit/1(direction) -> Product/2
  VPA Position/1 -> Sum/1
  Center of Mass/1 -> Sum/2
  Sum/1 -> Cross Product/1

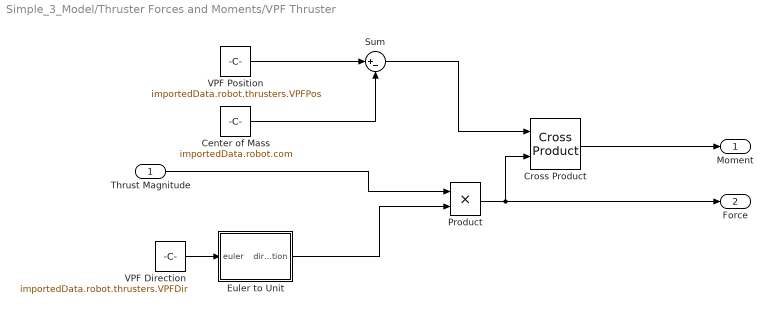
== system Simple_3_Model/Thruster Forces and Moments/VPF Thruster ==
  Thrust Magnitude : Inport
  Center of Mass : Constant  Value=importedData.robot.com
  Cross Product : matrix_library/Cross Product
      settings: SourceProductBaseCode=SL
  Euler to Unit : MATLAB Function  TreatAsAtomicUnit=on
  Product : Product
  Sum : Sum  Inputs=|+-
  VPF Direction : Constant  Value=importedData.robot.thrusters.VPFDir  VectorParams1D=off
  VPF Position : Constant  Value=importedData.robot.thrusters.VPFPos  VectorParams1D=off
  Moment : Outport
  Force : Outport  Port=2
  wires:
  Product/1 -> Force/1, Cross Product/2
  Cross Product/1 -> Moment/1
  Thrust Magnitude/1 -> Product/1
  VPF Direction/1 -> Euler to Unit/1(euler)
  Euler to Unit/1(direction) -> Product/2
  VPF Position/1 -> Sum/1
  Center of Mass/1 -> Sum/2
  Sum/1 -> Cross Product/1

== system Simple_3_Model/Thruster Forces and Moments/VSA Thruster ==
  Thrust Magnitude : Inport
  Center of Mass : Constant  Value=importedData.robot.com
  Cross Product : matrix_library/Cross Product
      settings: SourceProductBaseCode=SL
  Euler to Unit : MATLAB Function  TreatAsAtomicUnit=on
  Product : Product
  Sum : Sum  Inputs=|+-
  VSA Direction : Constant  Value=importedData.robot.thrusters.VSADir  VectorParams1D=off
  VSA Position : Constant  Value=importedData.robot.thrusters.VSAPos  VectorParams1D=off
  Moment : Outport
  Force : Outport  Port=2
  wires:
  Product/1 -> Force/1, Cross Product/2
  Cross Product/1 -> Moment/1
  Thrust Magnitude/1 -> Product/1
  VSA Direction/1 -> Euler to Unit/1(euler)
  Euler to Unit/1(direction) -> Product/2
  VSA Position/1 -> Sum/1
  Center of Mass/1 -> Sum/2
  Sum/1 -> Cross Product/1

== system Simple_3_Model/Thruster Forces and Moments/VSF Thruster ==
  Thrust Magnitude : Inport
  Center of Mass : Constant  Value=importedData.robot.com
  Cross Product : matrix_library/Cross Product
      settings: SourceProductBaseCode=SL
  Euler to Unit : MATLAB Function  TreatAsAtomicUnit=on
  Product : Product
  Sum : Sum  Inputs=|+-
  VSF Direction : Constant  Value=importedData.robot.thrusters.VSFDir  VectorParams1D=off
  VSF Position : Constant  Value=importedData.robot.thrusters.VSFPos  VectorParams1D=off
  Moment : Outport
  Force : Outport  Port=2
  wires:
  Product/1 -> Force/1, Cross Product/2
  Cross Product/1 -> Moment/1
  Thrust Magnitude/1 -> Product/1
  VSF Direction/1 -> Euler to Unit/1(euler)
  Euler to Unit/1(direction) -> Product/2
  VSF Position/1 -> Sum/1
  Center of Mass/1 -> Sum/2
  Sum/1 -> Cross Product/1

== matlab function Simple_3_Model/Linear Drag/Row to Column Vector ==
  data: row input; column output
function column = fcn(row)

column = [row(1); row(2); row(3)];

== matlab function Simple_3_Model/Thruster Forces and Moments/HSA Thruster/Euler to Unit ==
  data: euler input; direction output
function direction = fcn(euler)

directionCol = eul2rotm(euler, "XYZ") * [1; 0; 0];
direction = [directionCol(1,1), directionCol(2,1), directionCol(3,1)];

== matlab function Simple_3_Model/Thruster Forces and Moments/HPA Thruster/Euler to Unit ==
  data: euler input; direction output
function direction = fcn(euler)

directionCol = eul2rotm(euler, "XYZ") * [1; 0; 0];
direction = [directionCol(1,1), directionCol(2,1), directionCol(3,1)];

== matlab function Simple_3_Model/Thruster Forces and Moments/HPF Thruster/Euler to Unit ==
  data: euler input; direction output
function direction = fcn(euler)

directionCol = eul2rotm(euler, "XYZ") * [1; 0; 0];
direction = [directionCol(1,1), directionCol(2,1), directionCol(3,1)];

== matlab function Simple_3_Model/Thruster Forces and Moments/VSF Thruster/Euler to Unit ==
  data: euler input; direction output
function direction = fcn(euler)

directionCol = eul2rotm(euler, "XYZ") * [1; 0; 0];
direction = [directionCol(1,1), directionCol(2,1), directionCol(3,1)];

== matlab function Simple_3_Model/Thruster Forces and Moments/VSA Thruster/Euler to Unit ==
  data: euler input; direction output
function direction = fcn(euler)

directionCol = eul2rotm(euler, "XYZ") * [1; 0; 0];
direction = [directionCol(1,1), directionCol(2,1), directionCol(3,1)];

== matlab function Simple_3_Model/Thruster Forces and Moments/VPA Thruster/Euler to Unit ==
  data: euler input; direction output
function direction = fcn(euler)

directionCol = eul2rotm(euler, "XYZ") * [1; 0; 0];
direction = [directionCol(1,1), directionCol(2,1), directionCol(3,1)];

== matlab function Simple_3_Model/Thruster Forces and Moments/VPF Thruster/Euler to Unit ==
  data: euler input; direction output
function direction = fcn(euler)

directionCol = eul2rotm(euler, "XYZ") * [1; 0; 0];
direction = [directionCol(1,1), directionCol(2,1), directionCol(3,1)];

== matlab function Simple_3_Model/Buoyancy/Create Bouancy Vector ==
  data: magnitude input; bouyantForce output
function bouyantForce = fcn(magnitude)

bouyantForce = [0, 0, magnitude];

== matlab function Simple_3_Model/Gravity/Create Vector ==
  data: magnitude input; vector output
function vector = fcn(magnitude)

vector = [0, 0, magnitude];

== matlab function Simple_3_Model/Thruster Forces and Moments/To World Frame ==
  data: angularPosition input; rotation output
function rotation  = fcn(angularPosition)

rotationToRobot = eul2rotm([angularPosition(1,1), angularPosition(2,1), angularPosition(3,1)]); %create the rotation matrix to robot frame
rotation = inv(rotationToRobot);

== matlab function Simple_3_Model/Linear Drag/Create Rotation Matrix ==
  data: inverse output; angularPosition input; rotation output
function [inverse, rotation] = fcn(angularPosition)

initialCalculation = false; % doesnt add noise unless needed
rotation = zeros(3,3);
inverse = [nan, nan, nan; nan, nan, nan; nan, nan, nan];

%loop to find a rotation matrix that has a non-zero determinant
%while(sum(sum(isnan(inverse))) ~= 0)
%
%    if(initialCalculation)
%        disp("Singular Matrix Found -- Adding Noise!")
%        angularPosition = angularPosition + [rand() * 10^-5; rand() * 10^-5; rand() * 10^-5];
%    end
%
%    rotation = eul2rotm([angularPosition(1,1), angularPosition(2,1), angularPosition(3,1)]);
%    inverse = inv(rotation);
%
%    initialCalculation = true;
%end
rotation = eul2rotm([angularPosition(1,1), angularPosition(2,1), angularPosition(3,1)]);
inverse = inv(rotation);

== matlab function Simple_3_Model/Thruster Forces and Moments/Convert to Column Vector ==
  data: row input; column output
function column = fcn(row)

column = [row(1); row(2); row(3)];

== matlab function Simple_3_Model/Thruster Forces and Moments/Convert to Row Vector ==
  data: column input; row output
function row = fcn(column)

row = [column(1,1), column(2,1), column(3,1)];

== matlab function Simple_3_Model/Thruster Forces and Moments/Convert to Column Vector1 ==
  data: row input; column output
function column = fcn(row)

column = [row(1); row(2); row(3)];

== matlab function Simple_3_Model/Thruster Forces and Moments/Convert to Row Vector1 ==
  data: column input; row output
function row = fcn(column)

row = [column(1,1), column(2,1), column(3,1)];

== matlab function Simple_3_Model/Linear Drag/Seperate to Components ==
  data: x output; robotFrameVelocity input; y output; z output
function [x, y, z] = fcn(robotFrameVelocity)

x = robotFrameVelocity(1, 1);
y = robotFrameVelocity(2, 1);
z = robotFrameVelocity(3, 1);

== matlab function Simple_3_Model/Linear Drag/Concatenate Drag ==
  data: x input; velocityVector output; y input; z input
function velocityVector = fcn(x,y,z)

velocityVector = [x; y; z];

== matlab function Simple_3_Model/Linear Drag/Seperate to World Compents ==
  data: x output; robotFrameVelocity input; y output; z output
function [x, y, z] = fcn(robotFrameVelocity)

x = robotFrameVelocity(1, 1);
y = robotFrameVelocity(2, 1);
z = robotFrameVelocity(3, 1);

== matlab function Simple_3_Model/Angular Drag/Concatenate Drag ==
  data: roll input; velocityVector output; pitch input; yaw input
function velocityVector = fcn(roll,pitch,yaw)

velocityVector = [roll; pitch; yaw];

== matlab function Simple_3_Model/Angular Drag/Concatenate Velocity ==
  data: row input; column output
function column = fcn(row)

column = [row(1); row(2); row(3)];

== matlab function Simple_3_Model/Angular Drag/Create Rotation Matrix ==
  data: inverse output; angularPosition input; rotation output
function [inverse, rotation] = fcn(angularPosition)

rotation = eul2rotm([angularPosition(1,1), angularPosition(2,1), angularPosition(3,1)]);
inverse = inv(rotation);

== matlab function Simple_3_Model/Angular Drag/Seperate to Components ==
  data: roll output; pitch output; yaw output; robotFrameVelocity input
function [roll, pitch, yaw] = fcn(robotFrameVelocity)

roll = robotFrameVelocity(1, 1);
pitch = robotFrameVelocity(2, 1);
yaw = robotFrameVelocity(3, 1);

== matlab function Simple_3_Model/Angular Drag/Seperate to World Compents ==
  data: roll output; robotFrameVelocity input; pitch output; yaw output
function [roll, pitch, yaw] = fcn(robotFrameVelocity)

roll = robotFrameVelocity(1, 1);
pitch = robotFrameVelocity(2, 1);
yaw = robotFrameVelocity(3, 1);

== matlab function Simple_3_Model/Thruster Forces and Moments/HSF Thruster/Euler to Unit ==
  data: euler input; direction output
function direction = fcn(euler)

directionCol = eul2rotm(euler, "XYZ") * [1; 0; 0];
direction = [directionCol(1,1), directionCol(2,1), directionCol(3,1)];
